simulink model "ekf"  (R2023a)
settings: Solver=VariableStepAuto  StartTime=0.0  StopTime=30  RelTol=1e-3
model workspace (MAT data in the model file):
  Ts = 0.01
  a = 0.945
  b = 0.63
  theta = 0
  wf = 1.272
  wr = 1.21
libraries: sharedTrackingLibrary x1, fuzblock x1, simulink x1
settings Model: Creator=Jonat  LastModifiedBy=Jonat
settings DataIOCC: ReturnWorkspaceOutputs=off

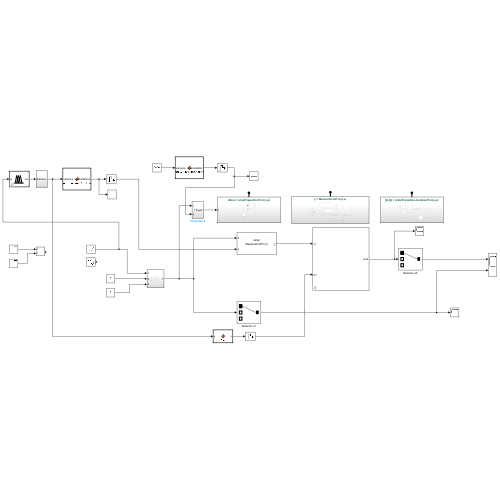
[thumbnail: Simulink's stored preview of the top-level diagram]
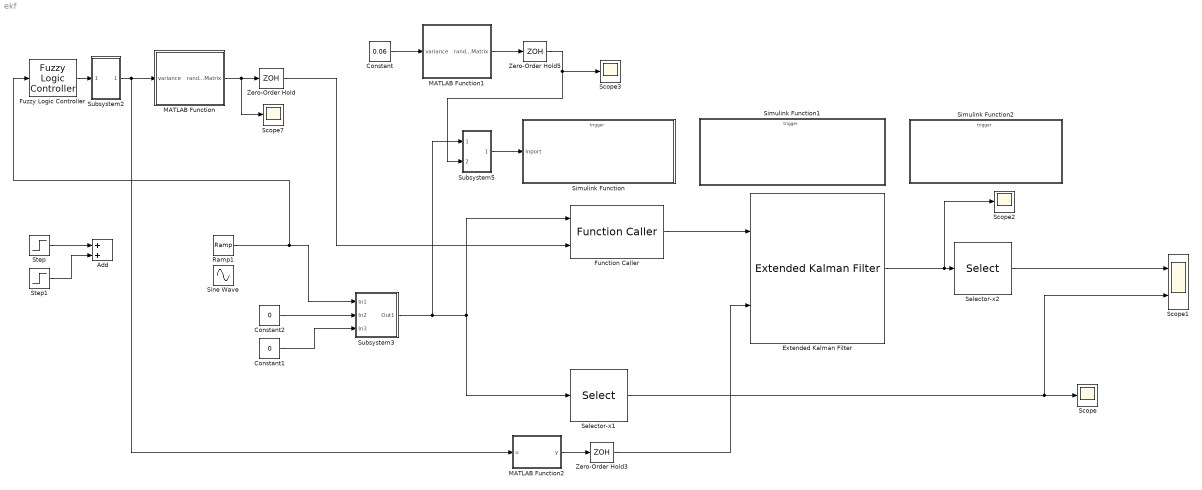
== system ekf ==
  Add : Sum
  Constant : Constant  Value=0.06
  Constant1 : Constant  Value=0
  Constant2 : Constant  Value=0
  Extended Kalman Filter : sharedTrackingLibrary/Extended Kalman Filter  StateTransitionFcn=stateTransitionFcn  HasStateTransitionJacobianFcn=on  StateTransitionJacobianFcn=stateTransitionJacobianFcn  HasAdditiveProcessNoise=Nonadditive  ProcessNoise=[0.05 0 0;0 0.05 0;0 0 0.002]  HasTimeVaryingProcessNoise=off  HasStateTransitionFcnExtraArgument=0  InitialState=[0; 0; 0]  InitialStateCovariance=10  MeasurementFcn1=MeasurmentFcn  HasMeasurementJacobianFcn1=off  HasMeasurementEnablePort1=off  HasAdditiveMeasurementNoise1=Nonadditive  MeasurementNoise1=[0.005 0 0 0;0 0.005 0 0;0 0 0.005 0;0 0 0 0.005]  HasTimeVaryingMeasurementNoise1=on  HasMeasurementFcnExtraArgument1=0  HasMeasurementWrapping1=off  MeasurementFcn2=myMeasurementFcn  HasMeasurementJacobianFcn2=off  HasMeasurementEnablePort2=off  HasAdditiveMeasurementNoise2=Additive  MeasurementNoise2=1  HasTimeVaryingMeasurementNoise2=off  HasMeasurementFcnExtraArgument2=0  HasMeasurementWrapping2=off  MeasurementFcn3=myMeasurementFcn  HasMeasurementJacobianFcn3=off  HasMeasurementEnablePort3=off  HasAdditiveMeasurementNoise3=Additive  MeasurementNoise3=1  HasTimeVaryingMeasurementNoise3=off  HasMeasurementFcnExtraArgument3=0  HasMeasurementWrapping3=off  MeasurementFcn4=myMeasurementFcn  HasMeasurementJacobianFcn4=off  HasMeasurementEnablePort4=off  HasAdditiveMeasurementNoise4=Additive  MeasurementNoise4=1  HasTimeVaryingMeasurementNoise4=off  HasMeasurementFcnExtraArgument4=0  HasMeasurementWrapping4=off  MeasurementFcn5=myMeasurementFcn  HasMeasurementJacobianFcn5=off  HasMeasurementEnablePort5=off  HasAdditiveMeasurementNoise5=Additive  MeasurementNoise5=1  HasTimeVaryingMeasurementNoise5=off  HasMeasurementFcnExtraArgument5=0  HasMeasurementWrapping5=off  EnableMultirate=off  StateTransitionFcnSampleTime=1  MeasurementFcn1SampleTime=1  MeasurementFcn2SampleTime=1  MeasurementFcn3SampleTime=1  MeasurementFcn4SampleTime=1  MeasurementFcn5SampleTime=1  UseCurrentEstimator=on  OutputStateCovariance=off  DataType=double  SampleTime=0.01  NumberOfMeasurements=1
      settings: LibrarySourceBlock=slident/Estimators/Extended Kalman Filter
  Function Caller : FunctionCaller  FunctionPrototype=y = MeasurmentFcn(x,v)  InputArgumentSpecifications=zeros(3,1), zeros(4,1)  OutputArgumentSpecifications=zeros(4,1)
  Fuzzy Logic Controller : fuzblock/Fuzzy Logic  Controller  FIS=for_ekf  OutputSampleNumber=101  DataType=double  FuzzifiedInputs=off  RuleFiringStrengths=off  RuleOutputs=off  AggregatedOutputs=off  SimulateUsing=Interpreted execution  OutOfRangeInputValueMessage=warning  NoRuleFiredMessage=warning  EmptyOutputFuzzySetMessage=warning
  MATLAB Function : MATLAB Function  TreatAsAtomicUnit=on
  MATLAB Function1 : MATLAB Function  TreatAsAtomicUnit=on
  MATLAB Function2 : MATLAB Function  TreatAsAtomicUnit=on
  Ramp1 : simulink/Sources/Ramp  slope=1  start=0  InitialOutput=0
  Scope{,2..3,7} (4 alike) : Scope
  Scope1 : Scope  NumInputPorts=2
  Selector-x1 : Selector  InputPortWidth=3  IndexOptions=Index vector (dialog)  Indices=[1]  OutputSizes=1
  Selector-x2 : Selector  InputPortWidth=3  IndexOptions=Index vector (dialog)  Indices=[1]  OutputSizes=1
  Simulink Function : Subsystem  TreatAsAtomicUnit=on
  Simulink Function1 : Subsystem  TreatAsAtomicUnit=on
  Simulink Function2 : Subsystem  TreatAsAtomicUnit=on
  Sine Wave : Sin  Amplitude=15  Frequency=0.4  SampleTime=0
  Step : Step  Time=5  After=15  SampleTime=0
  Step1 : Step  Time=15  Before=15  After=30  SampleTime=0
  Subsystem2 : Subsystem
  Subsystem3 : Subsystem
  Subsystem5 : Subsystem
  Zero-Order Hold : ZeroOrderHold  SampleTime=0.01
  Zero-Order Hold3 : ZeroOrderHold  SampleTime=0.01
  Zero-Order Hold5 : ZeroOrderHold  SampleTime=0.01
  wires:
  Selector-x1/1 -> Scope1/2, Scope/1
  Extended Kalman Filter/1 -> Scope2/1, Selector-x2/1
  Selector-x2/1 -> Scope1/1
  MATLAB Function/1(randomMatrix) -> Scope7/1, Zero-Order Hold/1
  Fuzzy Logic Controller/1 -> Subsystem2/1(In1)
  Subsystem3/1(Out1) -> Subsystem5/1(In1), Selector-x1/1, Function Caller/1
  Ramp1/1 -> Fuzzy Logic Controller/1, Subsystem3/1(In1)
  Constant1/1 -> Subsystem3/3(In3)
  Subsystem2/1(variance) -> MATLAB Function2/1(u), MATLAB Function/1(variance)
  Function Caller/1 -> Extended Kalman Filter/1
  MATLAB Function2/1(y) -> Zero-Order Hold3/1
  Zero-Order Hold3/1 -> Extended Kalman Filter/2
  Zero-Order Hold/1 -> Function Caller/2
  Subsystem5/1(Inport) -> Simulink Function/1(Inport)
  Constant/1 -> MATLAB Function1/1(variance)
  MATLAB Function1/1(randomMatrix) -> Zero-Order Hold5/1
  Zero-Order Hold5/1 -> Scope3/1, Subsystem5/2(In2)
  Constant2/1 -> Subsystem3/2(In2)
  Step/1 -> Add/1
  Step1/1 -> Add/2

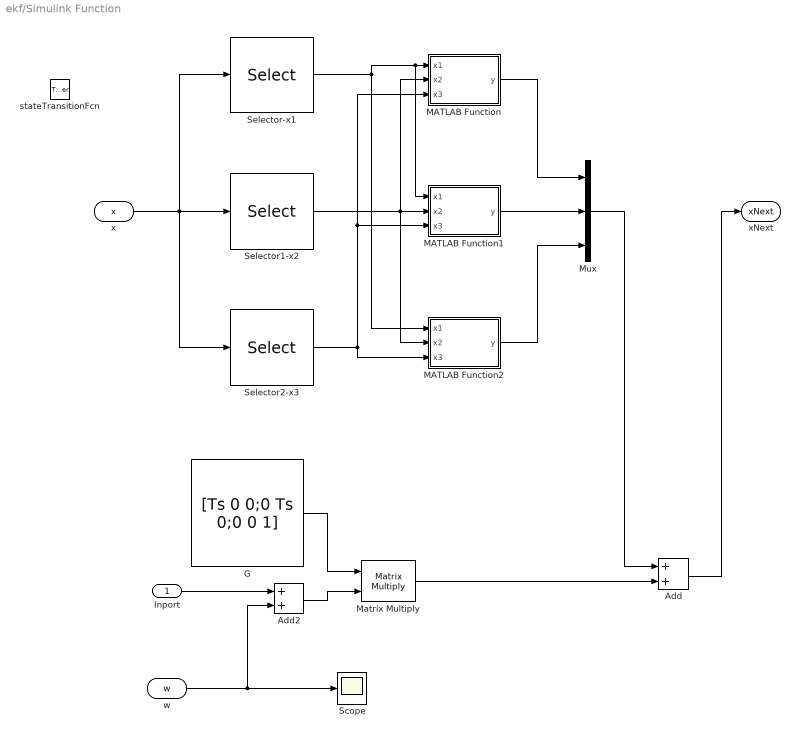
== system ekf/Simulink Function ==
  Inport : Inport  PortDimensions=3
  stateTransitionFcn : TriggerPort  TriggerType=function-call  IsSimulinkFunction=on  FunctionName=stateTransitionFcn  FunctionVisibility=scoped  VariantControl=(inherit)
  Add : Sum
  Add2 : Sum
  G : Constant  Value=[Ts 0 0;0 Ts 0;0 0 1]
  MATLAB Function : MATLAB Function  TreatAsAtomicUnit=on
  MATLAB Function1 : MATLAB Function  TreatAsAtomicUnit=on
  MATLAB Function2 : MATLAB Function  TreatAsAtomicUnit=on
  Matrix Multiply : Product  Multiplication=Matrix(*)
  Mux : Mux  Inputs=3
  Scope : Scope
  Selector-x1 : Selector  InputPortWidth=3  IndexOptions=Index vector (dialog)  Indices=[1]  OutputSizes=1
  Selector1-x2 : Selector  InputPortWidth=3  IndexOptions=Index vector (dialog)  Indices=[2]  OutputSizes=1
  Selector2-x3 : Selector  InputPortWidth=3  IndexOptions=Index vector (dialog)  Indices=[3]  OutputSizes=1
  x : ArgIn  DisableCoverage=on  PortDimensions=3  ArgumentName=x
  w : ArgIn  Port=2  PortDimensions=3  ArgumentName=w
  xNext : ArgOut  DisableCoverage=on  PortDimensions=3  ArgumentName=xNext
  wires:
  x/1 -> Selector2-x3/1, Selector1-x2/1, Selector-x1/1
  Selector-x1/1 -> MATLAB Function2/1(x1), MATLAB Function1/1(x1), MATLAB Function/1(x1)
  Selector1-x2/1 -> MATLAB Function1/2(x2), MATLAB Function/2(x2), MATLAB Function2/2(x2)
  Selector2-x3/1 -> MATLAB Function2/3(x3), MATLAB Function/3(x3), MATLAB Function1/3(x3)
  MATLAB Function/1(y) -> Mux/1
  MATLAB Function1/1(y) -> Mux/2
  MATLAB Function2/1(y) -> Mux/3
  G/1 -> Matrix Multiply/1
  Matrix Multiply/1 -> Add/2
  Mux/1 -> Add/1
  Inport/1 -> Add2/1
  Add/1 -> xNext/1
  w/1 -> Scope/1, Add2/2
  Add2/1 -> Matrix Multiply/2

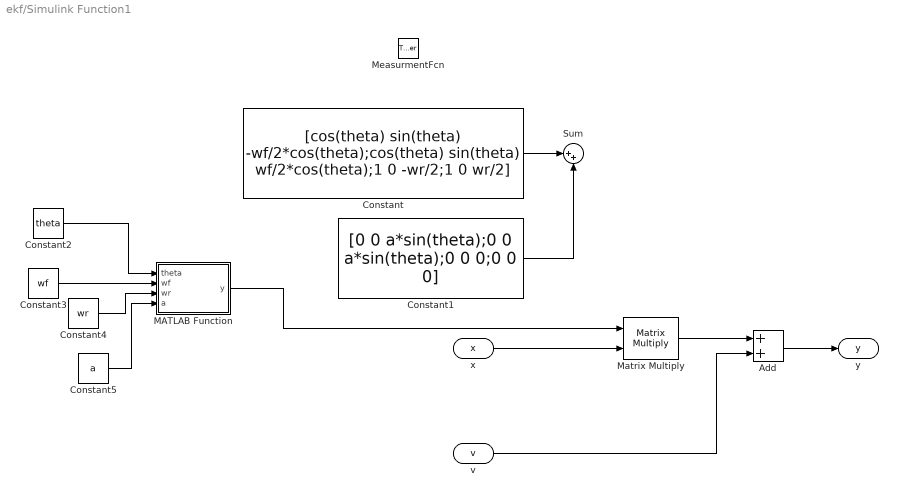
== system ekf/Simulink Function1 ==
  MeasurmentFcn : TriggerPort  TriggerType=function-call  IsSimulinkFunction=on  FunctionName=MeasurmentFcn  FunctionVisibility=scoped  VariantControl=(inherit)
  Add : Sum
  Constant : Constant  Value=[cos(theta) sin(theta) -wf/2*cos(theta);cos(theta) sin(theta) wf/2*cos(theta);1 0 -wr/2;1 0 wr/2]
  Constant1 : Constant  Value=[0 0 a*sin(theta);0 0 a*sin(theta);0 0 0;0 0 0]
  Constant2 : Constant  Value=theta
  Constant3 : Constant  Value=wf
  Constant4 : Constant  Value=wr
  Constant5 : Constant  Value=a
  MATLAB Function : MATLAB Function  TreatAsAtomicUnit=on
  Matrix Multiply : Product  Multiplication=Matrix(*)
  Sum : Sum  Inputs=|++
  x : ArgIn  DisableCoverage=on  PortDimensions=3  ArgumentName=x
  v : ArgIn  Port=2  PortDimensions=4  ArgumentName=v
  y : ArgOut  DisableCoverage=on  PortDimensions=4  ArgumentName=y
  wires:
  Constant/1 -> Sum/1
  Constant1/1 -> Sum/2
  x/1 -> Matrix Multiply/2
  Matrix Multiply/1 -> Add/1
  v/1 -> Add/2
  Add/1 -> y/1
  Constant3/1 -> MATLAB Function/2(wf)
  Constant5/1 -> MATLAB Function/4(a)
  Constant2/1 -> MATLAB Function/1(theta)
  Constant4/1 -> MATLAB Function/3(wr)
  MATLAB Function/1(y) -> Matrix Multiply/1

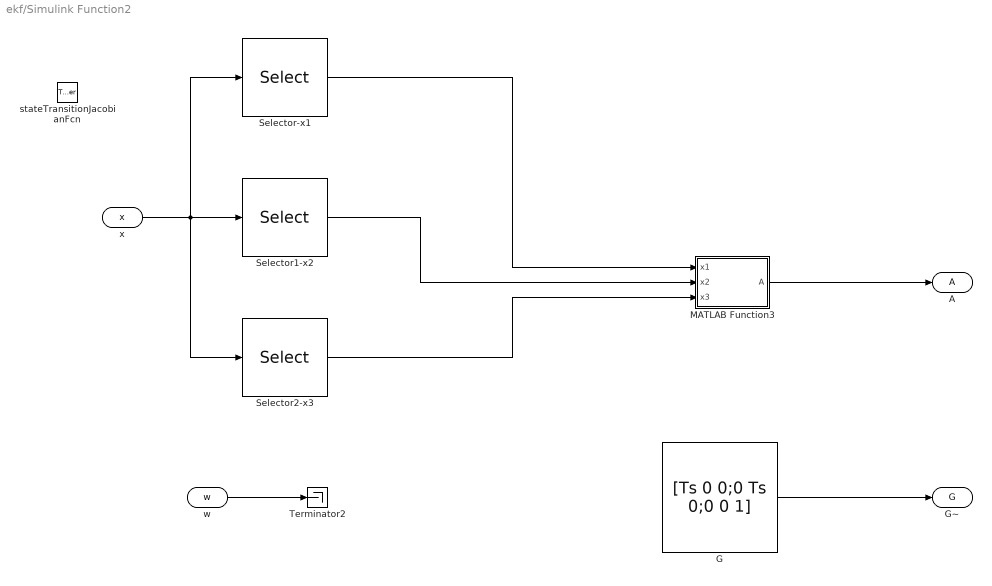
== system ekf/Simulink Function2 ==
  stateTransitionJacobianFcn : TriggerPort  TriggerType=function-call  IsSimulinkFunction=on  FunctionName=stateTransitionJacobianFcn  FunctionVisibility=scoped  VariantControl=(inherit)
  G : Constant  Value=[Ts 0 0;0 Ts 0;0 0 1]
  MATLAB Function3 : MATLAB Function  TreatAsAtomicUnit=on
  Selector-x1 : Selector  InputPortWidth=3  IndexOptions=Index vector (dialog)  Indices=[1]  OutputSizes=1
  Selector1-x2 : Selector  InputPortWidth=3  IndexOptions=Index vector (dialog)  Indices=[2]  OutputSizes=1
  Selector2-x3 : Selector  InputPortWidth=3  IndexOptions=Index vector (dialog)  Indices=[3]  OutputSizes=1
  Terminator2 : Terminator
  x : ArgIn  DisableCoverage=on  PortDimensions=3  ArgumentName=x
  w : ArgIn  Port=2  PortDimensions=3  ArgumentName=w
  A : ArgOut  DisableCoverage=on  PortDimensions=[3 3]  ArgumentName=A
  G~ : ArgOut  Port=2  PortDimensions=[3 3]  ArgumentName=G
  wires:
  x/1 -> Selector2-x3/1, Selector1-x2/1, Selector-x1/1
  w/1 -> Terminator2/1
  G/1 -> G~/1
  Selector-x1/1 -> MATLAB Function3/1(x1)
  Selector1-x2/1 -> MATLAB Function3/2(x2)
  Selector2-x3/1 -> MATLAB Function3/3(x3)
  MATLAB Function3/1(A) -> A/1

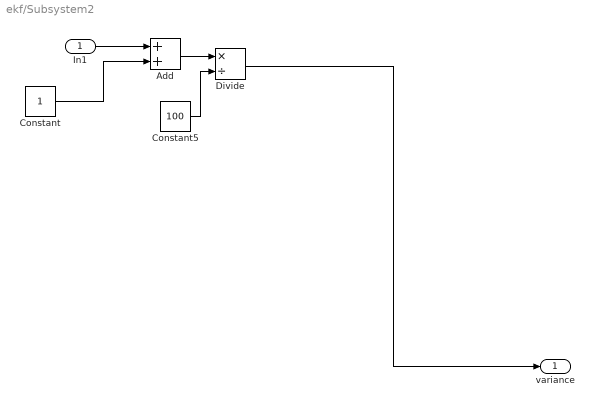
== system ekf/Subsystem2 ==
  In1 : Inport
  Add : Sum
  Constant : Constant
  Constant5 : Constant  Value=100
  Divide : Product  Inputs=*/
  variance : Outport
  wires:
  Add/1 -> Divide/1
  In1/1 -> Add/1
  Constant5/1 -> Divide/2
  Constant/1 -> Add/2
  Divide/1 -> variance/1

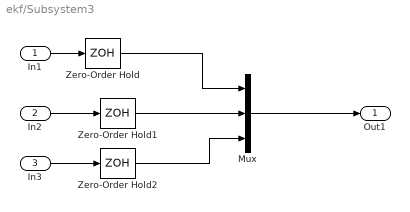
== system ekf/Subsystem3 ==
  In1 : Inport
  In2 : Inport  Port=2
  In3 : Inport  Port=3
  Mux : Mux  Inputs=3
  Zero-Order Hold : ZeroOrderHold  SampleTime=0.01
  Zero-Order Hold1 : ZeroOrderHold  SampleTime=0.01
  Zero-Order Hold2 : ZeroOrderHold  SampleTime=0.01
  Out1 : Outport
  wires:
  Zero-Order Hold2/1 -> Mux/3
  Zero-Order Hold1/1 -> Mux/2
  Mux/1 -> Out1/1
  Zero-Order Hold/1 -> Mux/1
  In3/1 -> Zero-Order Hold2/1
  In2/1 -> Zero-Order Hold1/1
  In1/1 -> Zero-Order Hold/1

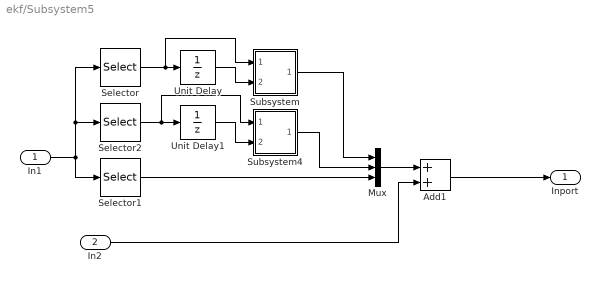
== system ekf/Subsystem5 ==
  In1 : Inport  PortDimensions=3
  In2 : Inport  Port=2  PortDimensions=3
  Add1 : Sum
  Mux : Mux  Inputs=3
  Selector : Selector  InputPortWidth=3  IndexOptions=Index vector (dialog)  Indices=[1]  OutputSizes=1
  Selector1 : Selector  InputPortWidth=3  IndexOptions=Index vector (dialog)  Indices=[3]  OutputSizes=1
  Selector2 : Selector  InputPortWidth=3  IndexOptions=Index vector (dialog)  Indices=[2]  OutputSizes=1
  Subsystem : Subsystem
  Subsystem4 : Subsystem
  Unit Delay : UnitDelay  SampleTime=-1  HasFrameUpgradeWarning=on
  Unit Delay1 : UnitDelay  SampleTime=-1  HasFrameUpgradeWarning=on
  Inport : Outport
  wires:
  In1/1 -> Selector2/1, Selector/1, Selector1/1
  Selector/1 -> Subsystem/1(In1), Unit Delay/1
  Subsystem/1(Out1) -> Mux/1
  Subsystem4/1(Out1) -> Mux/2
  Unit Delay/1 -> Subsystem/2(In2)
  Selector1/1 -> Mux/3
  Selector2/1 -> Subsystem4/1(In1), Unit Delay1/1
  Unit Delay1/1 -> Subsystem4/2(In2)
  Mux/1 -> Add1/1
  In2/1 -> Add1/2
  Add1/1 -> Inport/1

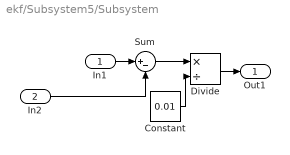
== system ekf/Subsystem5/Subsystem ==
  In1 : Inport
  In2 : Inport  Port=2
  Constant : Constant  Value=0.01
  Divide : Product  Inputs=*/
  Sum : Sum  Inputs=|+-
  Out1 : Outport
  wires:
  Constant/1 -> Divide/2
  Sum/1 -> Divide/1
  Divide/1 -> Out1/1
  In2/1 -> Sum/2
  In1/1 -> Sum/1

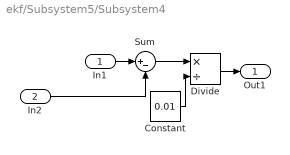
== system ekf/Subsystem5/Subsystem4 ==
  In1 : Inport
  In2 : Inport  Port=2
  Constant : Constant  Value=0.01
  Divide : Product  Inputs=*/
  Sum : Sum  Inputs=|+-
  Out1 : Outport
  wires:
  Constant/1 -> Divide/2
  Sum/1 -> Divide/1
  Divide/1 -> Out1/1
  In2/1 -> Sum/2
  In1/1 -> Sum/1

== matlab function ekf/Simulink Function/MATLAB Function1 ==
  data: x1 input; y output; x2 input; x3 input
function y = fcn(x1,x2,x3)

y = x2-0.01*x1*x3;

== matlab function ekf/Simulink Function/MATLAB Function ==
  data: x1 input; y output; x2 input; x3 input
function y = fcn(x1,x2,x3)

y = x1+0.01*x2*x3;

== matlab function ekf/Simulink Function/MATLAB Function2 ==
  data: x1 input; y output; x2 input; x3 input
function y = fcn(x1,x2,x3)

y = 0;

== matlab function ekf/MATLAB Function ==
  data: variance input; randomMatrix output
function randomMatrix = generateGaussianRandomMatrix(variance)
    % 生成具有高斯分布的4x1矩阵
    % 输入参数：
    %   variance: 方差
    % 输出参数：
    %   randomMatrix: 4x1矩阵

    % 使用 randn 函数生成高斯分布的随机值，并构建4x1矩阵
    randomValues = sqrt(variance) * randn(4, 1);

    % 将随机值存储为4x1矩阵
    randomMatrix = randomValues;
end

== matlab function ekf/MATLAB Function1 ==
  data: variance input; randomMatrix output
function randomMatrix = generateGaussianRandomMatrix(variance)
    % 生成具有高斯分布的4x1矩阵
    % 输入参数：
    %   variance: 方差
    % 输出参数：
    %   randomMatrix: 4x1矩阵

    % 使用 randn 函数生成高斯分布的随机值，并构建4x1矩阵
    randomValues = sqrt(variance) * randn(3, 1);

    % 将随机值存储为4x1矩阵
    randomMatrix = randomValues;
end

== matlab function ekf/Simulink Function1/MATLAB Function ==
  data: theta input; y output; wf input; wr input; a input
function y = fcn(theta,wf,wr,a)

y = [cos(theta) sin(theta) -wf/2*cos(theta)+a*sin(theta); cos(theta) sin(theta) wf/2*cos(theta)+a*sin(theta); 1 0 -wr/2; 1 0 wr/2];

== matlab function ekf/Simulink Function2/MATLAB Function3 ==
  data: x1 input; A output; x2 input; x3 input
function A = fcn(x1,x2,x3)


Ts=0.01;
A = [1 Ts*x3 Ts*x2; -Ts*x3 1 -Ts*x1; 0 0 0];

== matlab function ekf/MATLAB Function2 ==
  data: u input; y output
function y = fcn(u)
   
y = [u 0 0 0;
     0 u 0 0;
     0 0 u 0;
     0 0 0 u];
